simulink model "PCwF2M"  (R2015a)
settings: Solver=ode23  SolverMode=SingleTasking  StartTime=0.0  StopTime=50  RelTol=1e-7
values from neighbouring files (symbols this model uses):
  d1 = 100    [PCwF2Minit.m]
  d2 = 100    [PCwF2Minit.m]
  d3 = 100    [PCwF2Minit.m]
  d4 = 100    [PCwF2Minit.m]
  delta3 = 30    [PCwF2Minit.m]
  delta4 = 30    [PCwF2Minit.m]
  g = [0;0;-9.81]    [PCwF2Minit.m]
  H = blkdiag([eye(3) zeros(3)],[eye(3) zeros(3)])    [PCwF2Minit.m]
  j0 = 10    [PCwF2Minit.m]
  j1 = 10    [PCwF2Minit.m]
  j1d = 1.00*j1    (= 10)    [PCwF2Minit.m]
  j2 = 10    [PCwF2Minit.m]
  j2d = 1.00*j2    (= 10)    [PCwF2Minit.m]
  j3 = 10    [PCwF2Minit.m]
  j3d = 1.00*j3    (= 10)    [PCwF2Minit.m]
  j4 = 10    [PCwF2Minit.m]
  j4d = 1.00*j4    (= 10)    [PCwF2Minit.m]
  k1 = 50    [PCwF2Minit.m]
  k2 = 50    [PCwF2Minit.m]
  k3 = 5    [PCwF2Minit.m]
  k4 = 5    [PCwF2Minit.m]
  kappa3 = 50    [PCwF2Minit.m]
  kappa4 = 50    [PCwF2Minit.m]
  m0 = 10    [PCwF2Minit.m]
  m1 = 10    [PCwF2Minit.m]
  m1d = 1.00*m1    (= 10)    [PCwF2Minit.m]
  m2 = 10    [PCwF2Minit.m]
  m2d = 1.00*m2    (= 10)    [PCwF2Minit.m]
  m3 = 10    [PCwF2Minit.m]
  m3d = 1.00*m3    (= 10)    [PCwF2Minit.m]
  m4 = 10    [PCwF2Minit.m]
  m4d = 1.00*m4    (= 10)    [PCwF2Minit.m]
libraries: aerolibutil x5, dspinverses x3
settings Model: CovSFcnEnable=off  Creator=Martin  LastModifiedBy=mangerer
settings SolverCC: ZeroCrossAlgorithm=Adaptive
settings DataIOCC: LimitDataPoints=off
settings OptimizationCC: BlockReduction=off  BooleanDataType=off
settings DebuggingCC: SaveWithParameterizedLinksMsg=none  UnderspecifiedInitializationDetection=Classic  MergeDetectMultiDrivingBlocksExec=none  SignalResolutionControl=TryResolveAllWithWarning
settings HardwareCC: TargetUnknown=on

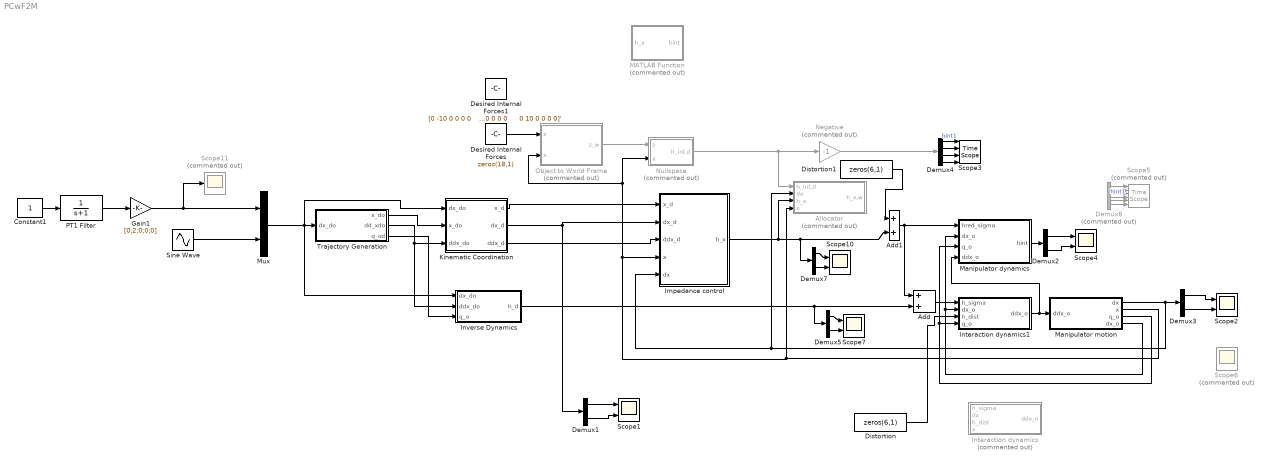
== system PCwF2M ==
  Add : Sum
  Add1 : Sum
  Allocator : Subsystem  Commented=on
  Constant1 : Constant
  Demux{1..3,5,7} (5 alike) : Demux  Outputs=2
  Demux4 : Demux
  Demux6 : Demux  Commented=on  Outputs=6
  Desired Internal Forces : Constant  Value=zeros(18,1)
  Desired Internal Forces1 : Constant  Value="[0 -10 0 0 0 0    10 0 0 0 0 0      0 10 0 0 0 0]'"
  Distortion : Constant  Value=zeros(6,1)
  Distortion1 : Constant  Value=zeros(6,1)
  Gain1 : Gain  Gain=[0;2;0;0;0]
  Impedance control : Subsystem
  Interaction dynamics : Subsystem  Commented=on
  Interaction dynamics1 : Subsystem
  Inverse Dynamics : Subsystem
  Kinematic Coordination : Subsystem
  MATLAB Function : MATLAB Function  Commented=on  TreatAsAtomicUnit=on
  Manipulator dynamics : Subsystem
  Manipulator motion : Subsystem
  Mux : Mux  Inputs=2
  Negative : Gain  Commented=on  Gain=-1
  Nullspace : Subsystem  Commented=on
  Object to World Frame : MATLAB Function  Commented=on  TreatAsAtomicUnit=on
  PT1 Filter : TransferFcn  Denominator=[1 1]
  Scope{1..2,4,7,10} (5 alike) : Scope  NumInputPorts=2
      Scope1 settings: ShowLegends=on  YMin=-1~-1  YMax=1~1
      Scope10 settings: ShowLegends=on  YMin=-75~-75  YMax=75~75  SaveName=ScopeData18
      Scope2 settings: ShowLegends=on  YMin=-0.25~-0.25  YMax=3~3  SaveName=ScopeData2
      Scope4 settings: ShowLegends=on  YMin=-0.2~-0.2  YMax=0.2~0.2  SaveName=ScopeData5
      Scope7 settings: ShowLegends=on  YMin=-75~-75  YMax=75~75  SaveName=ScopeData7
  Scope11 : Scope  Commented=on
      settings: YMin=0.9984  YMax=1  SaveName=ScopeData26
  Scope3 : TimeScope  NumInputPorts=4
  Scope5 : TimeScope  Commented=on  NumInputPorts=6
  Scope6 : Scope  Commented=on  NumInputPorts=4
      settings: ShowLegends=on  YMin=-25~-25~-25~-25  YMax=200~200~200~200  SaveName=ScopeData11
  Sine Wave : Sin  Frequency=2*pi  SampleTime=0
  Trajectory Generation : Subsystem
  wires:
  Manipulator dynamics/1(hint) -> Demux2/1
  Demux2/2 -> Scope4/2
  Demux3/1 -> Scope2/1
  Demux3/2 -> Scope2/2
  Add1/1 -> Manipulator dynamics/1(hred_sigma), Add/1
  Object to World Frame/1(z_w) -> Nullspace/1(z)
  Nullspace/1(h_int,d) -> Negative/1, Allocator/1(h_int,d)
  Demux7/1 -> Scope10/1
  Demux7/2 -> Scope10/2
  PT1 Filter/1 -> Gain1/1
  Gain1/1 -> Mux/1, Scope11/1
  Impedance control/1(h_x) -> Allocator/3(h_x), Add1/2, Demux7/1
  Manipulator motion/1(dx) -> Impedance control/5(dx), Allocator/2(dx), Demux3/1
  Trajectory Generation/2(dd_xdo) -> Inverse Dynamics/2(ddx_do), Kinematic Coordination/3(ddx_do)
  Mux/1 -> Inverse Dynamics/1(dx_do), Kinematic Coordination/1(dx_do), Trajectory Generation/1(dx_do)
  Kinematic Coordination/1(x_d) -> Impedance control/1(x_d)
  Kinematic Coordination/3(ddx_d) -> Impedance control/3(ddx_d)
  Manipulator motion/2(x) -> Object to World Frame/2(x), Nullspace/2(x), Impedance control/4(x), Allocator/4(x)
  Constant1/1 -> PT1 Filter/1
  Demux1/1 -> Scope1/1
  Demux1/2 -> Scope1/2
  Kinematic Coordination/2(dx_d) -> Impedance control/2(dx_d), Demux1/1
  Negative/1 -> Demux4/1
  Demux4/1 -> Scope3/1  "hint1"
  Demux4/2 -> Scope3/2
  Demux4/4 -> Scope3/4
  Sine Wave/1 -> Mux/2
  Demux6/1 -> Scope5/1  "hint1"
  Demux6/2 -> Scope5/2
  Demux6/3 -> Scope5/3
  Demux6/4 -> Scope5/4
  Demux6/5 -> Scope5/5
  Demux6/6 -> Scope5/6
  Demux4/3 -> Scope3/3
  Desired Internal Forces/1 -> Object to World Frame/1(z)
  Add/1 -> Interaction dynamics1/1(h_sigma)
  Interaction dynamics1/1(ddx_o) -> Manipulator dynamics/4(ddx_o), Manipulator motion/1(ddx_o)
  Distortion/1 -> Interaction dynamics1/3(h_dist)
  Manipulator motion/3(q_o) -> Interaction dynamics1/4(q_o), Manipulator dynamics/3(q_o)
  Manipulator motion/4(dx_o) -> Interaction dynamics1/2(dx_o), Manipulator dynamics/2(dx_o)
  Distortion1/1 -> Add1/1
  Demux2/1 -> Scope4/1
  Demux5/1 -> Scope7/1
  Demux5/2 -> Scope7/2
  Inverse Dynamics/1(h_d) -> Demux5/1, Add/2
  Trajectory Generation/1(x_do) -> Kinematic Coordination/2(x_do)
  Trajectory Generation/3(q_od) -> Inverse Dynamics/3(q_o)

== system PCwF2M/Allocator ==
  h_int,d : Inport
  dx : Inport  Port=2
  h_x : Inport  Port=3
  x : Inport  Port=4
  Add : Sum  Inputs=-+
  Add1 : Sum
  Divide : Product  Inputs=*/*  Multiplication=Matrix(*)
  Divide1 : Product  Inputs=*/*  Multiplication=Matrix(*)
  Divide2 : Product  Inputs=*/*  Multiplication=Matrix(*)
  Inertia : Constant  Value=blkdiag(m1d*eye(3), j1d*eye(3), m2d*eye(3), j2d*eye(3), m3d*eye(3), j3d*eye(3), m4d*eye(3), j4d*eye(3))
  MATLAB Function : MATLAB Function  TreatAsAtomicUnit=on
  MATLAB Function1 : MATLAB Function  TreatAsAtomicUnit=on
  Math Function : Math  Operator=transpose  SaturateOnIntegerOverflow=on
  h_x,w : Outport
  wires:
  dx/1 -> MATLAB Function1/1(dx)
  Divide/1 -> h_x,w/1
  Math Function/1 -> Divide1/3, Divide/1
  MATLAB Function/1(Ared) -> Math Function/1, Divide2/1, Divide1/1
  Divide1/1 -> Divide/2
  Inertia/1 -> Divide1/2, Divide2/2
  MATLAB Function1/1(bred) -> Add/2
  Add/1 -> Divide/3
  Divide2/1 -> Add/1
  Add1/1 -> Divide2/3
  h_int,d/1 -> Add1/1
  h_x/1 -> Add1/2
  x/1 -> MATLAB Function1/2(x), MATLAB Function/1(x)

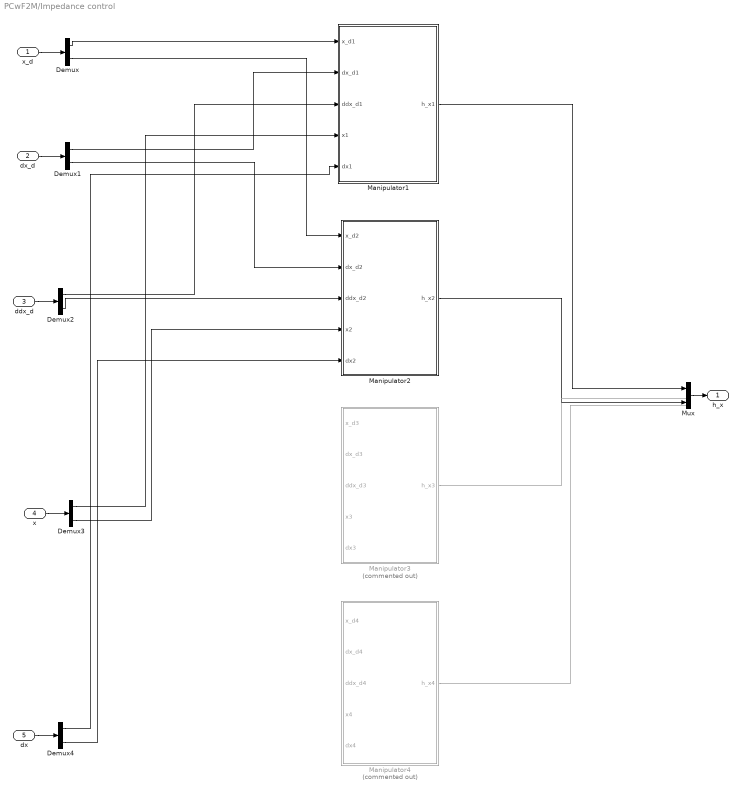
== system PCwF2M/Impedance control ==
  x_d : Inport
  dx_d : Inport  Port=2
  ddx_d : Inport  Port=3
  x : Inport  Port=4
  dx : Inport  Port=5
  Demux{,1..4} (5 alike) : Demux  Outputs=2
  Manipulator1 : Subsystem
  Manipulator2 : Subsystem
  Manipulator3 : Subsystem  Commented=on
  Manipulator4 : Subsystem  Commented=on
  Mux : Mux  Inputs=2
  h_x : Outport
  wires:
  dx/1 -> Demux4/1
  x/1 -> Demux3/1
  ddx_d/1 -> Demux2/1
  dx_d/1 -> Demux1/1
  x_d/1 -> Demux/1
  Demux/1 -> Manipulator1/1(x_d1)
  Demux/2 -> Manipulator2/1(x_d2)
  ? -> Manipulator3/1(x_d3)
  ? -> Manipulator4/1(x_d4)
  Demux1/1 -> Manipulator1/2(dx_d1)
  Demux1/2 -> Manipulator2/2(dx_d2)
  ? -> Manipulator3/2(dx_d3)
  ? -> Manipulator4/2(dx_d4)
  Demux2/1 -> Manipulator1/3(ddx_d1)
  Demux2/2 -> Manipulator2/3(ddx_d2)
  ? -> Manipulator3/3(ddx_d3)
  ? -> Manipulator4/3(ddx_d4)
  Demux3/1 -> Manipulator1/4(x1)
  Demux3/2 -> Manipulator2/4(x2)
  ? -> Manipulator3/4(x3)
  ? -> Manipulator4/4(x4)
  ? -> Manipulator4/5(dx4)
  ? -> Manipulator3/5(dx3)
  Demux4/2 -> Manipulator2/5(dx2)
  Demux4/1 -> Manipulator1/5(dx1)
  Mux/1 -> h_x/1
  Manipulator1/1(h_x1) -> Mux/1
  Manipulator2/1(h_x2) -> Mux/2
  Manipulator3/1(h_x3) -> ?
  Manipulator4/1(h_x4) -> ?

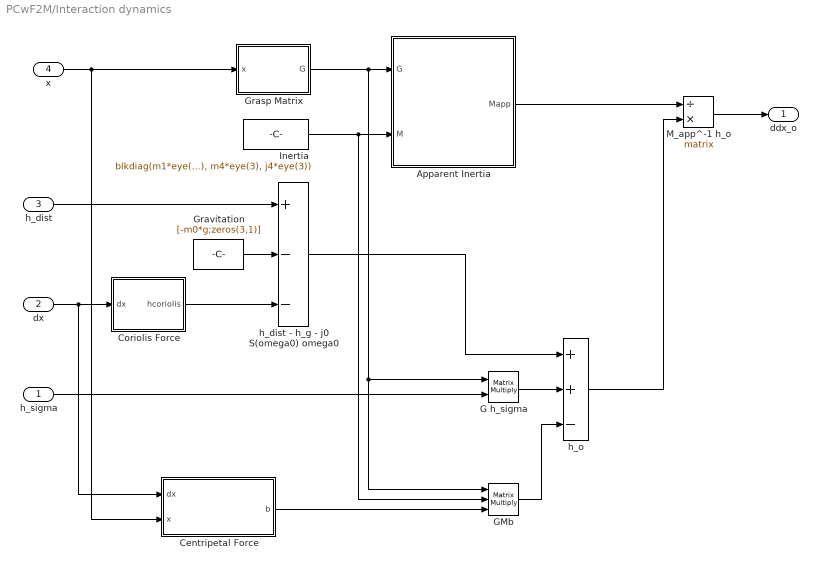
== system PCwF2M/Interaction dynamics ==
  h_sigma : Inport
  dx : Inport  Port=2
  h_dist : Inport  Port=3
  x : Inport  Port=4
  Apparent Inertia : MATLAB Function  TreatAsAtomicUnit=on
  Centripetal Force : MATLAB Function  TreatAsAtomicUnit=on
  Coriolis Force : MATLAB Function  TreatAsAtomicUnit=on
  G h_sigma : Product  Multiplication=Matrix(*)
  GMb : Product  Inputs=***  Multiplication=Matrix(*)
  Grasp Matrix : MATLAB Function  TreatAsAtomicUnit=on
  Gravitation : Constant  Value=[-m0*g;zeros(3,1)]
  Inertia : Constant  Value=blkdiag(m1*eye(3), j1*eye(3), m2*eye(3), j2*eye(3), m3*eye(3), j3*eye(3), m4*eye(3), j4*eye(3))
  M_app^-1 h_o : Product  Inputs=/*  Multiplication=Matrix(*)
  "h_dist - h_g - j0 S(omega0) omega0 " : Sum  Inputs=+--
  h_o : Sum  Inputs=++-
  ddx_o : Outport
  wires:
  Grasp Matrix/1(G) -> G h_sigma/1, GMb/1, Apparent Inertia/1(G)
  Inertia/1 -> GMb/2, Apparent Inertia/2(M)
  Apparent Inertia/1(Mapp) -> M_app^-1 h_o/1
  h_o/1 -> M_app^-1 h_o/2
  G h_sigma/1 -> h_o/2
  h_sigma/1 -> G h_sigma/2
  "h_dist - h_g - j0 S(omega0) omega0 "/1 -> h_o/1
  h_dist/1 -> "h_dist - h_g - j0 S(omega0) omega0 "/1
  Gravitation/1 -> "h_dist - h_g - j0 S(omega0) omega0 "/2
  dx/1 -> Centripetal Force/1(dx), Coriolis Force/1(dx)
  Coriolis Force/1(hcoriolis) -> "h_dist - h_g - j0 S(omega0) omega0 "/3
  GMb/1 -> h_o/3
  Centripetal Force/1(b) -> GMb/3
  M_app^-1 h_o/1 -> ddx_o/1
  x/1 -> Centripetal Force/2(x), Grasp Matrix/1(x)

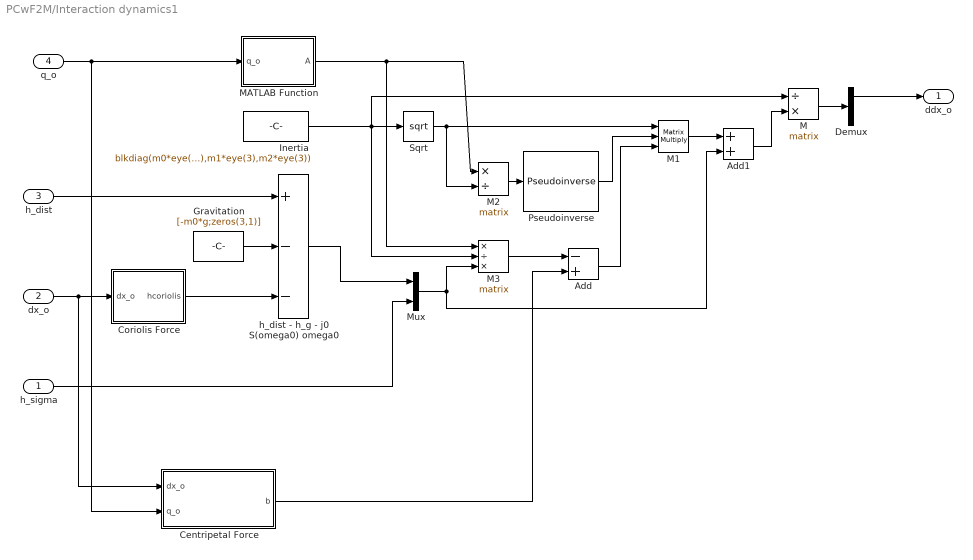
== system PCwF2M/Interaction dynamics1 ==
  h_sigma : Inport
  dx_o : Inport  Port=2
  h_dist : Inport  Port=3
  q_o : Inport  Port=4
  Add : Sum  Inputs=-+
  Add1 : Sum
  Centripetal Force : MATLAB Function  TreatAsAtomicUnit=on
  Coriolis Force : MATLAB Function  TreatAsAtomicUnit=on
  Demux : Demux  Outputs=2
  Gravitation : Constant  Value=[-m0*g;zeros(3,1)]
  Inertia : Constant  Value=blkdiag(m0*eye(3),j0*eye(3),m1*eye(3),m2*eye(3))
  M : Product  Inputs=/*  Multiplication=Matrix(*)
  M1 : Product  Inputs=***  Multiplication=Matrix(*)
  M2 : Product  Inputs=*/  Multiplication=Matrix(*)
  M3 : Product  Inputs=*/*  Multiplication=Matrix(*)
  MATLAB Function : MATLAB Function  TreatAsAtomicUnit=on
  Mux : Mux  Inputs=2
  Pseudoinverse : dspinverses/Pseudoinverse  wanterr=off
  Sqrt : Sqrt  SaturateOnIntegerOverflow=on
  "h_dist - h_g - j0 S(omega0) omega0 " : Sum  Inputs=+--
  ddx_o : Outport
  wires:
  h_dist/1 -> "h_dist - h_g - j0 S(omega0) omega0 "/1
  Gravitation/1 -> "h_dist - h_g - j0 S(omega0) omega0 "/2
  dx_o/1 -> Centripetal Force/1(dx_o), Coriolis Force/1(dx_o)
  Coriolis Force/1(hcoriolis) -> "h_dist - h_g - j0 S(omega0) omega0 "/3
  q_o/1 -> MATLAB Function/1(q_o), Centripetal Force/2(q_o)
  Inertia/1 -> M/1, M3/2, Sqrt/1
  Sqrt/1 -> M2/2, M1/1
  MATLAB Function/1(A) -> M3/1, M2/1
  M2/1 -> Pseudoinverse/1
  Pseudoinverse/1 -> M1/2
  Add/1 -> M1/3
  Centripetal Force/1(b) -> Add/2
  M3/1 -> Add/1
  Mux/1 -> Add1/2, M3/3
  "h_dist - h_g - j0 S(omega0) omega0 "/1 -> Mux/1
  h_sigma/1 -> Mux/2
  M/1 -> Demux/1
  Demux/1 -> ddx_o/1
  M1/1 -> Add1/1
  Add1/1 -> M/2

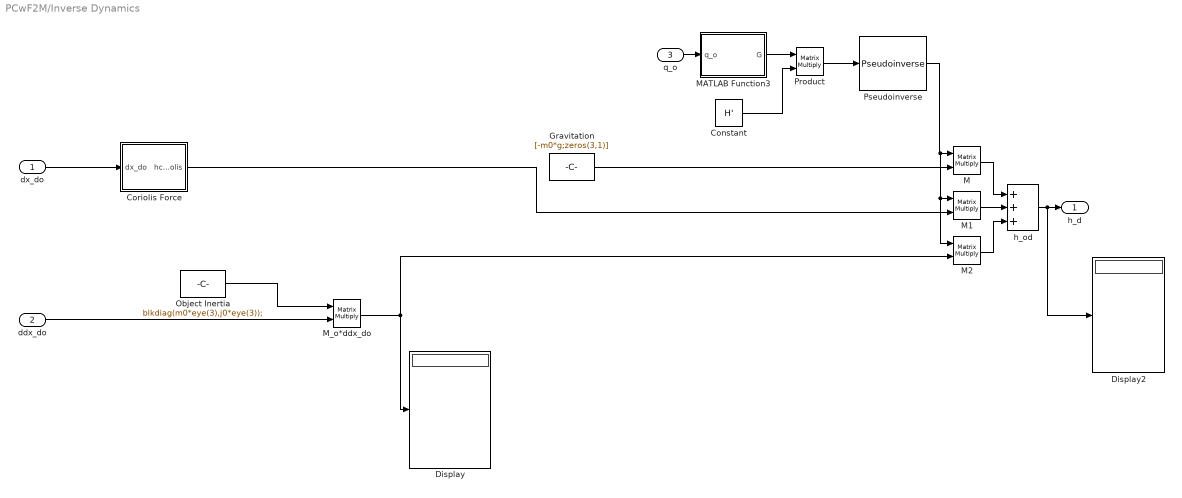
== system PCwF2M/Inverse Dynamics ==
  dx_do : Inport
  ddx_do : Inport  Port=2
  q_o : Inport  Port=3
  Constant : Constant  Value=H'
  Coriolis Force : MATLAB Function  TreatAsAtomicUnit=on
  Display : Display
  Display2 : Display
  Gravitation : Constant  Value=[-m0*g;zeros(3,1)]
  M : Product  Multiplication=Matrix(*)
  M1 : Product  Multiplication=Matrix(*)
  M2 : Product  Multiplication=Matrix(*)
  MATLAB Function3 : MATLAB Function  TreatAsAtomicUnit=on
  M_o*ddx_do : Product  Multiplication=Matrix(*)
  Object Inertia : Constant  Value=blkdiag(m0*eye(3),j0*eye(3));
  Product : Product  Multiplication=Matrix(*)
  Pseudoinverse : dspinverses/Pseudoinverse  wanterr=off
  h_od : Sum  Inputs=+++
  h_d : Outport
  wires:
  ddx_do/1 -> M_o*ddx_do/2
  Object Inertia/1 -> M_o*ddx_do/1
  dx_do/1 -> Coriolis Force/1(dx_do)
  q_o/1 -> MATLAB Function3/1(q_o)
  M_o*ddx_do/1 -> Display/1, M2/2
  Coriolis Force/1(hcoriolis) -> M1/2
  Pseudoinverse/1 -> M2/1, M1/1, M/1
  MATLAB Function3/1(G) -> Product/1
  Product/1 -> Pseudoinverse/1
  Constant/1 -> Product/2
  M1/1 -> h_od/2
  M/1 -> h_od/1
  M2/1 -> h_od/3
  h_od/1 -> Display2/1, h_d/1
  Gravitation/1 -> M/2

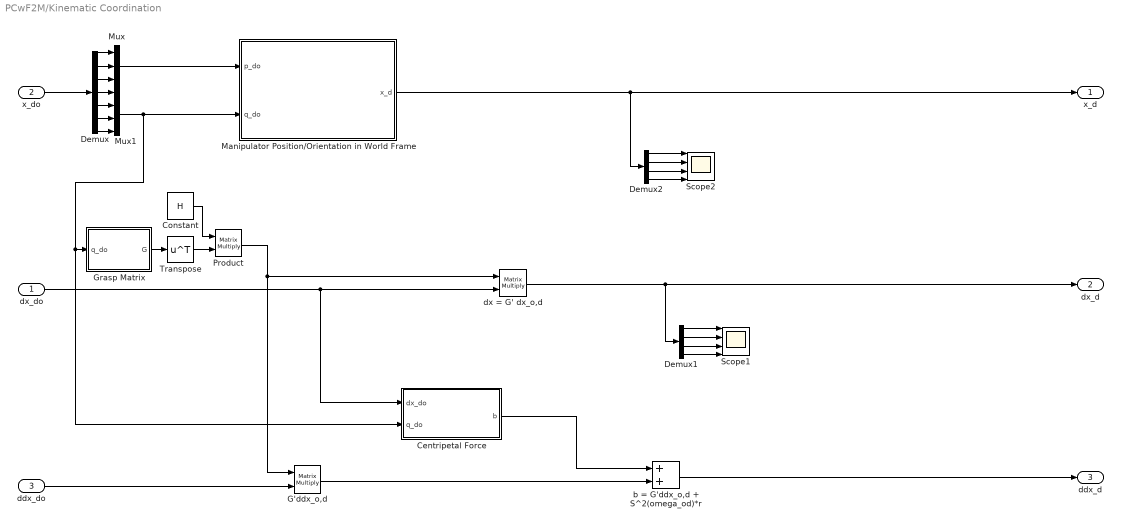
== system PCwF2M/Kinematic Coordination ==
  dx_do : Inport
  x_do : Inport  Port=2
  ddx_do : Inport  Port=3
  Centripetal Force : MATLAB Function  TreatAsAtomicUnit=on
  Constant : Constant  Value=H
  Demux : Demux  Outputs=7
  Demux1 : Demux
  Demux2 : Demux
  G'ddx_o,d : Product  Multiplication=Matrix(*)
  Grasp Matrix : MATLAB Function  TreatAsAtomicUnit=on
  Manipulator Position/Orientation in World Frame : MATLAB Function  TreatAsAtomicUnit=on
  Mux : Mux  Inputs=3
  Mux1 : Mux
  Product : Product  Multiplication=Matrix(*)
  Scope1 : Scope  NumInputPorts=4
      settings: ShowLegends=on  YMin=-1.5~-1.5~-1.5~-1.5  YMax=6~5.5~6~5.5  SaveName=ScopeData3
  Scope2 : Scope  NumInputPorts=4
      settings: ShowLegends=on  YMin=-1.5~-1.5~-1.5~-1.5  YMax=6~5.5~6~5.5  SaveName=ScopeData4
  Transpose : Math  Operator=transpose  SaturateOnIntegerOverflow=on
  b = G'ddx_o,d + S^2(omega_od)*r : Sum
  dx = G' dx_o,d : Product  Multiplication=Matrix(*)
  x_d : Outport
  dx_d : Outport  Port=2
  ddx_d : Outport  Port=3
  wires:
  Grasp Matrix/1(G) -> Transpose/1
  dx = G' dx_o,d/1 -> Demux1/1, dx_d/1
  x_do/1 -> Demux/1
  Demux/1 -> Mux/1
  Demux/2 -> Mux/2
  Demux/3 -> Mux/3
  Demux/5 -> Mux1/2
  Demux/6 -> Mux1/3
  Demux/7 -> Mux1/4
  Demux/4 -> Mux1/1
  Mux/1 -> Manipulator Position/Orientation in World Frame/1(p_do)
  Centripetal Force/1(b) -> b = G'ddx_o,d + S^2(omega_od)*r/1
  ddx_do/1 -> G'ddx_o,d/2
  G'ddx_o,d/1 -> b = G'ddx_o,d + S^2(omega_od)*r/2
  b = G'ddx_o,d + S^2(omega_od)*r/1 -> ddx_d/1
  dx_do/1 -> Centripetal Force/1(dx_do), dx = G' dx_o,d/2
  Demux1/1 -> Scope1/1
  Demux1/2 -> Scope1/2
  Demux1/3 -> Scope1/3
  Demux1/4 -> Scope1/4
  Manipulator Position/Orientation in World Frame/1(x_d) -> Demux2/1, x_d/1
  Demux2/1 -> Scope2/1
  Demux2/2 -> Scope2/2
  Demux2/3 -> Scope2/3
  Demux2/4 -> Scope2/4
  Transpose/1 -> Product/2
  Product/1 -> dx = G' dx_o,d/1, G'ddx_o,d/1
  Constant/1 -> Product/1
  Mux1/1 -> Centripetal Force/2(q_do), Grasp Matrix/1(q_do), Manipulator Position/Orientation in World Frame/2(q_do)

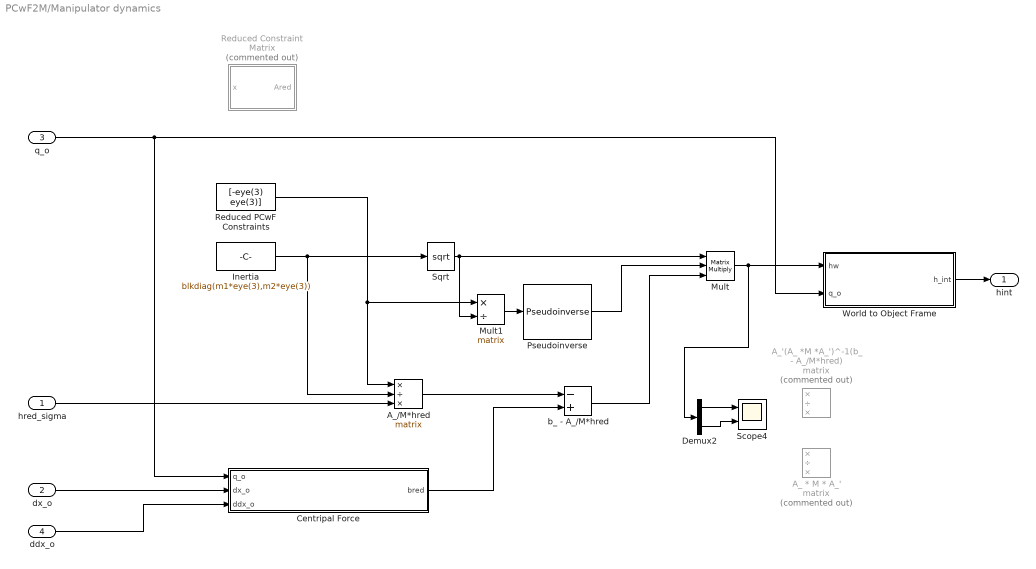
== system PCwF2M/Manipulator dynamics ==
  hred_sigma : Inport
  dx_o : Inport  Port=2
  q_o : Inport  Port=3
  ddx_o : Inport  Port=4
  A_ * M * A_' : Product  Commented=on  Inputs=*/*  Multiplication=Matrix(*)
  A_'(A_ *M *A_')^-1(b_ - A_/M*hred) : Product  Commented=on  Inputs=*/*  Multiplication=Matrix(*)
  A_/M*hred : Product  Inputs=*/*  Multiplication=Matrix(*)
  Centripal Force : MATLAB Function  TreatAsAtomicUnit=on
  Demux2 : Demux  Outputs=2
  Inertia : Constant  Value=blkdiag(m1*eye(3),m2*eye(3))
  Mult : Product  Inputs=***  Multiplication=Matrix(*)
  Mult1 : Product  Inputs=*/  Multiplication=Matrix(*)
  Pseudoinverse : dspinverses/Pseudoinverse  wanterr=off
  Reduced Constraint Matrix : MATLAB Function  Commented=on  TreatAsAtomicUnit=on
  Reduced PCwF Constraints : Constant  Value=[-eye(3) eye(3)]
  Scope4 : Scope  NumInputPorts=2
      settings: ShowLegends=on  YMin=-0.2~-0.175  YMax=0.175~0.2  SaveName=ScopeData8
  Sqrt : Sqrt  SaturateOnIntegerOverflow=on
  World to Object Frame : MATLAB Function  TreatAsAtomicUnit=on
  b_ - A_/M*hred : Sum  Inputs=-+
  hint : Outport
  wires:
  Inertia/1 -> Sqrt/1, A_/M*hred/2
  A_/M*hred/1 -> b_ - A_/M*hred/1
  hred_sigma/1 -> A_/M*hred/3
  World to Object Frame/1(h_int) -> hint/1
  q_o/1 -> Centripal Force/1(q_o), World to Object Frame/2(q_o)
  Centripal Force/1(bred) -> b_ - A_/M*hred/2
  b_ - A_/M*hred/1 -> Mult/3
  Sqrt/1 -> Mult1/2, Mult/1
  Mult1/1 -> Pseudoinverse/1
  Pseudoinverse/1 -> Mult/2
  Reduced PCwF Constraints/1 -> A_/M*hred/1, Mult1/1
  dx_o/1 -> Centripal Force/2(dx_o)
  ddx_o/1 -> Centripal Force/3(ddx_o)
  Mult/1 -> Demux2/1, World to Object Frame/1(hw)
  Demux2/2 -> Scope4/2
  Demux2/1 -> Scope4/1

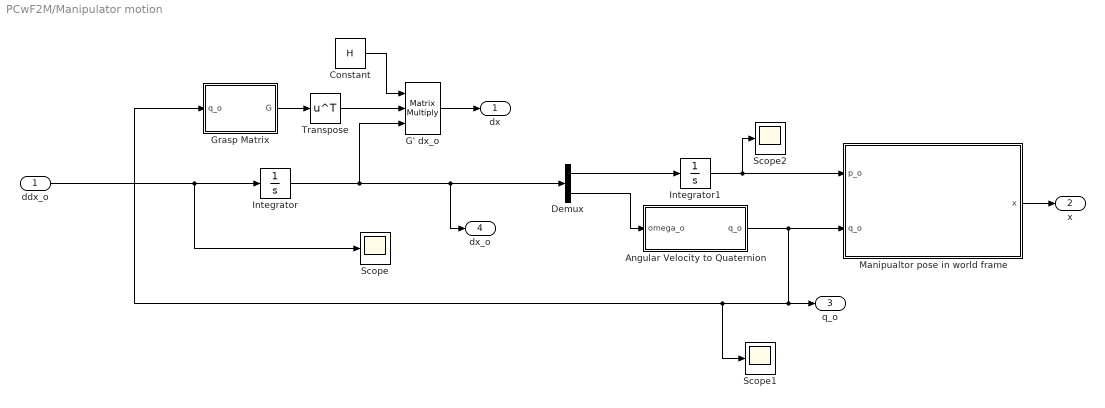
== system PCwF2M/Manipulator motion ==
  ddx_o : Inport
  Angular Velocity to Quaternion : Subsystem
  Constant : Constant  Value=H
  Demux : Demux  Outputs=2
  G' dx_o : Product  Inputs=3  Multiplication=Matrix(*)
  Grasp Matrix : MATLAB Function  TreatAsAtomicUnit=on
  Integrator : Integrator  InitialCondition=zeros(6,1)
  Integrator1 : Integrator  InitialCondition=[0 0 0]'
  Manipualtor pose in world frame : MATLAB Function  TreatAsAtomicUnit=on
  Scope : Scope
      settings: ShowLegends=on  YMin=-3.5  YMax=3.5  SaveName=ScopeData14
  Scope1 : Scope
      settings: YMin=-0.5  YMax=1  SaveName=ScopeData12
  Scope2 : Scope
      settings: ShowLegends=on  YMin=-10  YMax=150  SaveName=ScopeData6
  Transpose : Math  Operator=transpose  SaturateOnIntegerOverflow=on
  dx : Outport
  x : Outport  Port=2
  q_o : Outport  Port=3
  dx_o : Outport  Port=4
  wires:
  ddx_o/1 -> Scope/1, Integrator/1
  Integrator/1 -> G' dx_o/3, dx_o/1, Demux/1
  Grasp Matrix/1(G) -> Transpose/1
  G' dx_o/1 -> dx/1
  Demux/2 -> Angular Velocity to Quaternion/1(omega_o)
  Demux/1 -> Integrator1/1
  Integrator1/1 -> Scope2/1, Manipualtor pose in world frame/1(p_o)
  Manipualtor pose in world frame/1(x) -> x/1
  Angular Velocity to Quaternion/1(q_o) -> Scope1/1, Grasp Matrix/1(q_o), q_o/1, Manipualtor pose in world frame/2(q_o)
  Transpose/1 -> G' dx_o/2
  Constant/1 -> G' dx_o/1

== system PCwF2M/Nullspace ==
  z : Inport
  x : Inport  Port=2
  A_' * z : Product  Multiplication=Matrix(*)
  Reduced Constraint Matrix : MATLAB Function  TreatAsAtomicUnit=on
  Transpose : Math  Operator=transpose  SaturateOnIntegerOverflow=on
  h_int,d : Outport
  wires:
  Reduced Constraint Matrix/1(Ared) -> Transpose/1
  Transpose/1 -> A_' * z/1
  z/1 -> A_' * z/2
  A_' * z/1 -> h_int,d/1
  x/1 -> Reduced Constraint Matrix/1(x)

== system PCwF2M/Trajectory Generation ==
  dx_do : Inport
  Angular Velocity to Quaternion Orientation : Subsystem
  Demux : Demux  Outputs=2
  Demux1 : Demux  Outputs=7
  Derivative : Derivative
  Integrator : Integrator  InitialCondition=zeros(3,1)
  Mux : Mux  Inputs=2
  Mux1 : Mux  Inputs=3
  Mux2 : Mux
  Mux3 : Mux  Inputs=2
  Quaternion Normalize : aerolibutil/Quaternion Normalize
  x_do : Outport
  dd_xdo : Outport  Port=2
  q_od : Outport  Port=3
  wires:
  dx_do/1 -> Derivative/1, Demux/1
  Demux/2 -> Angular Velocity to Quaternion Orientation/1(omega_do)
  Demux/1 -> Integrator/1
  Angular Velocity to Quaternion Orientation/1(q_do) -> Quaternion Normalize/1
  Integrator/1 -> Mux/1
  Derivative/1 -> dd_xdo/1
  Quaternion Normalize/1 -> Mux/2
  Demux1/1 -> Mux1/1
  Demux1/2 -> Mux1/2
  Demux1/3 -> Mux1/3
  Demux1/4 -> Mux2/1
  Demux1/5 -> Mux2/2
  Demux1/6 -> Mux2/3
  Demux1/7 -> Mux2/4
  Mux/1 -> Demux1/1
  Mux1/1 -> Mux3/1
  Mux3/1 -> x_do/1
  Mux2/1 -> q_od/1, Mux3/2

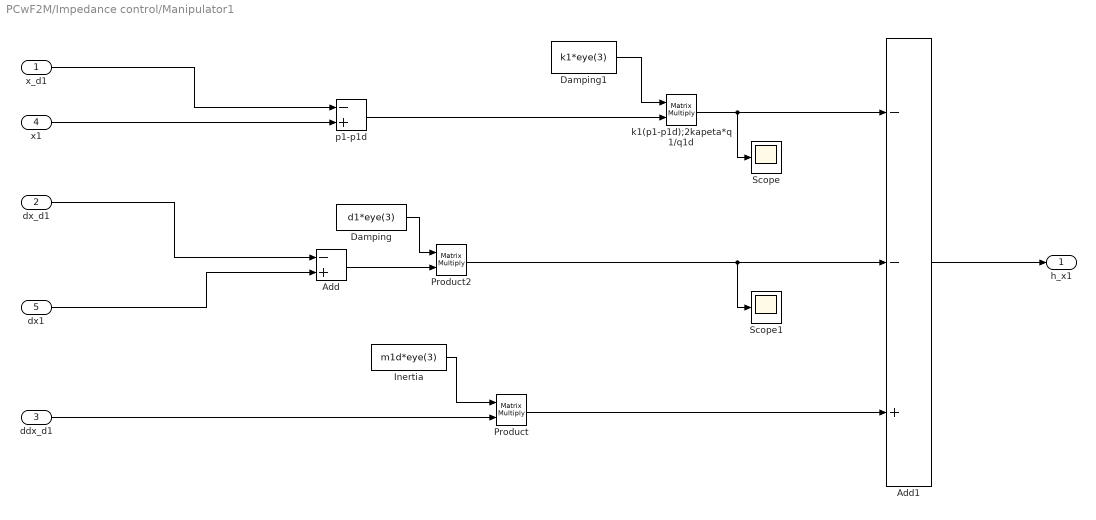
== system PCwF2M/Impedance control/Manipulator1 ==
  x_d1 : Inport
  dx_d1 : Inport  Port=2
  ddx_d1 : Inport  Port=3
  x1 : Inport  Port=4
  dx1 : Inport  Port=5
  Add : Sum  Inputs=-+
  Add1 : Sum  Inputs=--+
  Damping : Constant  Value=d1*eye(3)
  Damping1 : Constant  Value=k1*eye(3)
  Inertia : Constant  Value=m1d*eye(3)
  Product : Product  Multiplication=Matrix(*)
  Product2 : Product  Multiplication=Matrix(*)
  Scope : Scope
      settings: TimeRange=200  YMin=-50  YMax=125  SaveName=ScopeData13
  Scope1 : Scope
      settings: TimeRange=200  YMin=-50  YMax=125  SaveName=ScopeData19
  k1(p1-p1d);2kapeta*q1/q1d : Product  Multiplication=Matrix(*)
  p1-p1d : Sum  Inputs=-+
  h_x1 : Outport
  wires:
  Add/1 -> Product2/2
  Damping/1 -> Product2/1
  dx_d1/1 -> Add/1
  dx1/1 -> Add/2
  Inertia/1 -> Product/1
  Add1/1 -> h_x1/1
  k1(p1-p1d);2kapeta*q1/q1d/1 -> Scope/1, Add1/1
  Product2/1 -> Scope1/1, Add1/2
  Product/1 -> Add1/3
  ddx_d1/1 -> Product/2
  Damping1/1 -> k1(p1-p1d);2kapeta*q1/q1d/1
  p1-p1d/1 -> k1(p1-p1d);2kapeta*q1/q1d/2
  x_d1/1 -> p1-p1d/1
  x1/1 -> p1-p1d/2

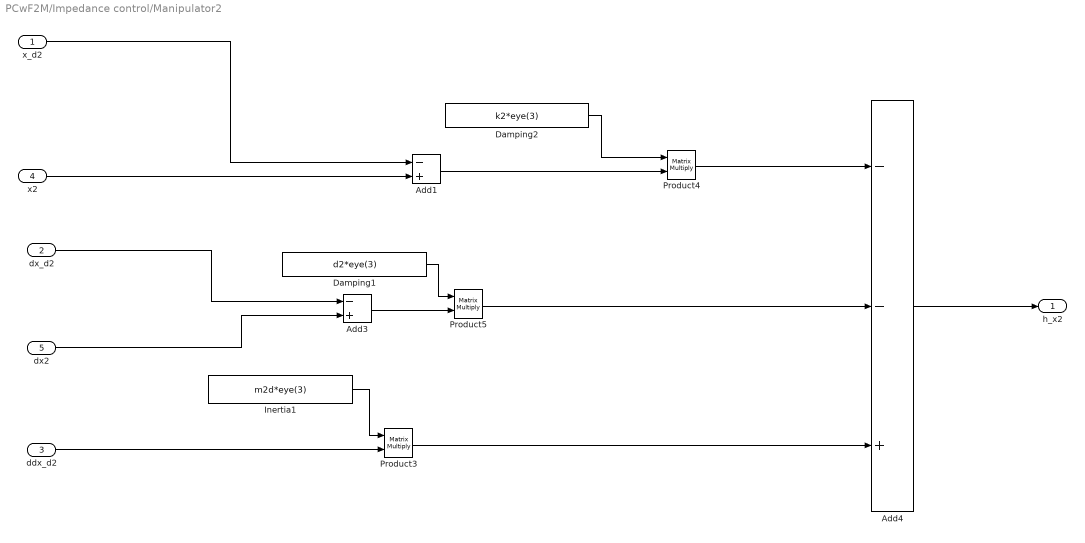
== system PCwF2M/Impedance control/Manipulator2 ==
  x_d2 : Inport
  dx_d2 : Inport  Port=2
  ddx_d2 : Inport  Port=3
  x2 : Inport  Port=4
  dx2 : Inport  Port=5
  Add1 : Sum  Inputs=-+
  Add3 : Sum  Inputs=-+
  Add4 : Sum  Inputs=--+
  Damping1 : Constant  Value=d2*eye(3)
  Damping2 : Constant  Value=k2*eye(3)
  Inertia1 : Constant  Value=m2d*eye(3)
  Product3 : Product  Multiplication=Matrix(*)
  Product4 : Product  Multiplication=Matrix(*)
  Product5 : Product  Multiplication=Matrix(*)
  h_x2 : Outport
  wires:
  Add3/1 -> Product5/2
  Damping1/1 -> Product5/1
  dx_d2/1 -> Add3/1
  dx2/1 -> Add3/2
  Inertia1/1 -> Product3/1
  Add4/1 -> h_x2/1
  Product4/1 -> Add4/1
  Product5/1 -> Add4/2
  Product3/1 -> Add4/3
  ddx_d2/1 -> Product3/2
  Damping2/1 -> Product4/1
  x_d2/1 -> Add1/1
  Add1/1 -> Product4/2
  x2/1 -> Add1/2

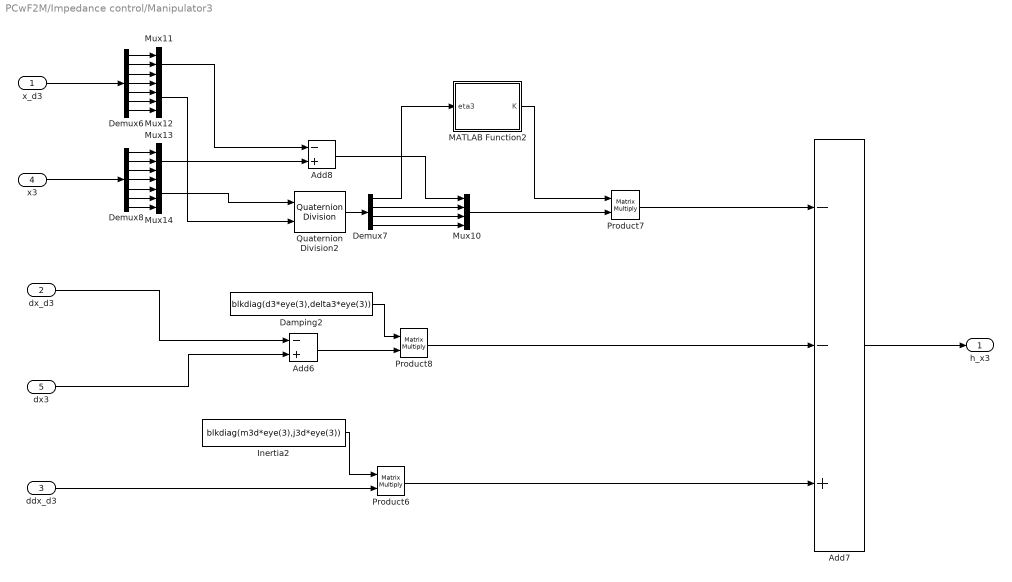
== system PCwF2M/Impedance control/Manipulator3 ==
  x_d3 : Inport
  dx_d3 : Inport  Port=2
  ddx_d3 : Inport  Port=3
  x3 : Inport  Port=4
  dx3 : Inport  Port=5
  Add6 : Sum  Inputs=-+
  Add7 : Sum  Inputs=--+
  Add8 : Sum  Inputs=-+
  Damping2 : Constant  Value=blkdiag(d3*eye(3),delta3*eye(3))
  Demux6 : Demux  Outputs=7
  Demux7 : Demux
  Demux8 : Demux  Outputs=7
  Inertia2 : Constant  Value=blkdiag(m3d*eye(3),j3d*eye(3))
  MATLAB Function2 : MATLAB Function  TreatAsAtomicUnit=on
  Mux10 : Mux
  Mux11 : Mux  Inputs=3
  Mux12 : Mux
  Mux13 : Mux  Inputs=3
  Mux14 : Mux
  Product6 : Product  Multiplication=Matrix(*)
  Product7 : Product  Multiplication=Matrix(*)
  Product8 : Product  Multiplication=Matrix(*)
  Quaternion Division2 : aerolibutil/Quaternion Division
  h_x3 : Outport
  wires:
  Add6/1 -> Product8/2
  Damping2/1 -> Product8/1
  dx_d3/1 -> Add6/1
  dx3/1 -> Add6/2
  MATLAB Function2/1(K) -> Product7/1
  Demux7/1 -> MATLAB Function2/1(eta3)
  Add8/1 -> Mux10/1
  Demux7/2 -> Mux10/2
  Demux7/3 -> Mux10/3
  Demux7/4 -> Mux10/4
  x3/1 -> Demux8/1
  x_d3/1 -> Demux6/1
  Demux6/2 -> Mux11/2
  Demux6/1 -> Mux11/1
  Demux6/3 -> Mux11/3
  Demux6/4 -> Mux12/1
  Demux6/5 -> Mux12/2
  Demux6/6 -> Mux12/3
  Demux6/7 -> Mux12/4
  Demux8/2 -> Mux13/2
  Demux8/1 -> Mux13/1
  Demux8/3 -> Mux13/3
  Demux8/4 -> Mux14/1
  Demux8/5 -> Mux14/2
  Demux8/6 -> Mux14/3
  Demux8/7 -> Mux14/4
  Mux11/1 -> Add8/1
  Mux13/1 -> Add8/2
  Quaternion Division2/1 -> Demux7/1
  Mux10/1 -> Product7/2
  Inertia2/1 -> Product6/1
  Add7/1 -> h_x3/1
  Product7/1 -> Add7/1
  Product8/1 -> Add7/2
  Product6/1 -> Add7/3
  ddx_d3/1 -> Product6/2
  Mux14/1 -> Quaternion Division2/1
  Mux12/1 -> Quaternion Division2/2

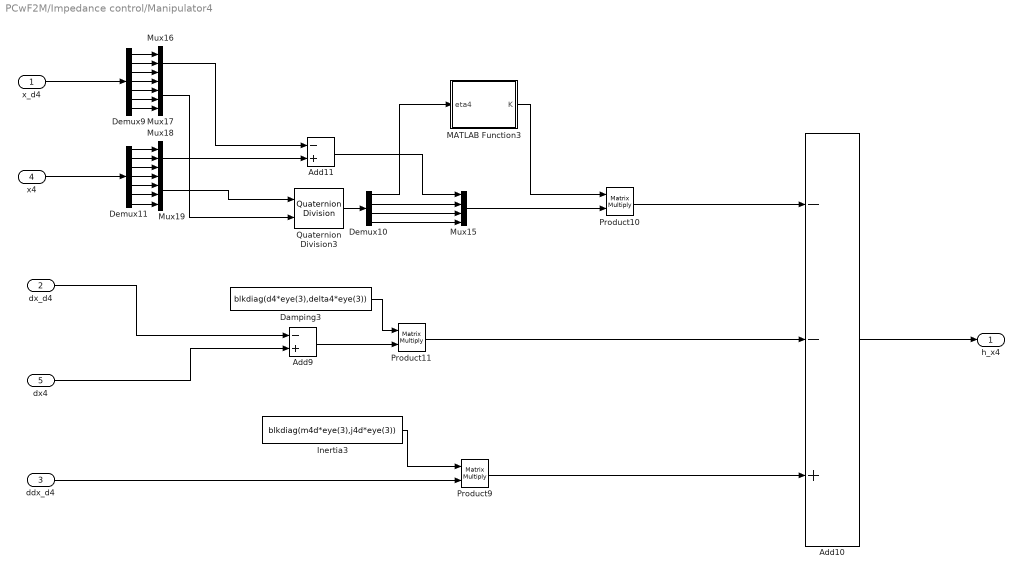
== system PCwF2M/Impedance control/Manipulator4 ==
  x_d4 : Inport
  dx_d4 : Inport  Port=2
  ddx_d4 : Inport  Port=3
  x4 : Inport  Port=4
  dx4 : Inport  Port=5
  Add10 : Sum  Inputs=--+
  Add11 : Sum  Inputs=-+
  Add9 : Sum  Inputs=-+
  Damping3 : Constant  Value=blkdiag(d4*eye(3),delta4*eye(3))
  Demux10 : Demux
  Demux11 : Demux  Outputs=7
  Demux9 : Demux  Outputs=7
  Inertia3 : Constant  Value=blkdiag(m4d*eye(3),j4d*eye(3))
  MATLAB Function3 : MATLAB Function  TreatAsAtomicUnit=on
  Mux15 : Mux
  Mux16 : Mux  Inputs=3
  Mux17 : Mux
  Mux18 : Mux  Inputs=3
  Mux19 : Mux
  Product10 : Product  Multiplication=Matrix(*)
  Product11 : Product  Multiplication=Matrix(*)
  Product9 : Product  Multiplication=Matrix(*)
  Quaternion Division3 : aerolibutil/Quaternion Division
  h_x4 : Outport
  wires:
  Add9/1 -> Product11/2
  Damping3/1 -> Product11/1
  dx_d4/1 -> Add9/1
  dx4/1 -> Add9/2
  MATLAB Function3/1(K) -> Product10/1
  Demux10/1 -> MATLAB Function3/1(eta4)
  Add11/1 -> Mux15/1
  Demux10/2 -> Mux15/2
  Demux10/3 -> Mux15/3
  Demux10/4 -> Mux15/4
  x4/1 -> Demux11/1
  x_d4/1 -> Demux9/1
  Demux9/2 -> Mux16/2
  Demux9/1 -> Mux16/1
  Demux9/3 -> Mux16/3
  Demux9/4 -> Mux17/1
  Demux9/5 -> Mux17/2
  Demux9/6 -> Mux17/3
  Demux9/7 -> Mux17/4
  Demux11/2 -> Mux18/2
  Demux11/1 -> Mux18/1
  Demux11/3 -> Mux18/3
  Demux11/4 -> Mux19/1
  Demux11/5 -> Mux19/2
  Demux11/6 -> Mux19/3
  Demux11/7 -> Mux19/4
  Mux16/1 -> Add11/1
  Mux18/1 -> Add11/2
  Quaternion Division3/1 -> Demux10/1
  Mux15/1 -> Product10/2
  Inertia3/1 -> Product9/1
  Add10/1 -> h_x4/1
  Product10/1 -> Add10/1
  Product11/1 -> Add10/2
  Product9/1 -> Add10/3
  ddx_d4/1 -> Product9/2
  Mux19/1 -> Quaternion Division3/1
  Mux17/1 -> Quaternion Division3/2

== system PCwF2M/Manipulator motion/Angular Velocity to Quaternion ==
  omega_o : Inport
  Constant : Constant  Value=0
  Gain : Gain  Gain=0.5
  Integrator : Integrator  InitialCondition=[1; 0; 0; 0]
  Mux : Mux  Inputs=2
  Quaternion Multiplication : aerolibutil/Quaternion Multiplication
  Scope : Scope
      settings: ShowLegends=on  SaveName=ScopeData9
  q_o : Outport
  wires:
  omega_o/1 -> Gain/1
  Gain/1 -> Mux/2
  Constant/1 -> Mux/1
  Quaternion Multiplication/1 -> Integrator/1
  Integrator/1 -> Quaternion Multiplication/2, q_o/1, Scope/1
  Mux/1 -> Quaternion Multiplication/1

== system PCwF2M/Trajectory Generation/Angular Velocity to Quaternion Orientation ==
  omega_do : Inport
  Constant : Constant  Value=0
  Gain : Gain  Gain=0.5
  Integrator : Integrator  InitialCondition=[1; 0; 0; 0]
  Mux : Mux  Inputs=2
  Quaternion Multiplication : aerolibutil/Quaternion Multiplication
  Scope : Scope
      settings: ShowLegends=on  SaveName=ScopeData9
  q_do : Outport
  wires:
  omega_do/1 -> Gain/1
  Gain/1 -> Mux/2
  Constant/1 -> Mux/1
  Quaternion Multiplication/1 -> Integrator/1
  Integrator/1 -> Quaternion Multiplication/2, Scope/1, q_do/1
  Mux/1 -> Quaternion Multiplication/1

== matlab function PCwF2M/Inverse Dynamics/Coriolis Force ==
  data: dx_do input; hcoriolis output; j0 parameter; m0 parameter
function hcoriolis = CoriolisForce(dx_do,j0,m0)
hcoriolis = [m0*skew_sm(dx_do(4:6))*dx_do(1:3);
        j0*skew_sm(dx_do(4:6))*dx_do(4:6)];

== matlab function PCwF2M/Interaction dynamics1/MATLAB Function ==
  data: r parameter; A output; q_o input
function A = ConstraintMatrix(r,q_o)
% A = [-eye(3) skew_sm(quatrot(x(4:7),r(1:3))) eye(3) zeros(3,21);
%         zeros(3) -eye(3) zeros(3) eye(3) zeros(3,18);
%         -eye(3) skew_sm(quatrot(x(4:7),r(4:6))) zeros(3,6) eye(3) zeros(3,15);
%         zeros(3) -eye(3) zeros(3,9) eye(3) zeros(3,12);
%         -eye(3) skew_sm(quatrot(x(4:7),r(7:9))) zeros(3,12) eye(3) zeros(3,9);
%         zeros(3) -eye(3) zeros(3,15) eye(3) zeros(3,6);
%         -eye(3) skew_sm(quatrot(x(4:7),r(10:12))) zeros(3,18) eye(3) zeros(3);
%         zeros(3) -eye(3) zeros(3,21) eye(3)];
A = [-eye(3) skew_sm(quatrot(q_o,r(1:3))) eye(3) zeros(3);
     -eye(3) skew_sm(quatrot(q_o,r(4:6))) zeros(3) eye(3)];

== matlab function PCwF2M/Interaction dynamics1/Centripetal Force ==
  data: dx_o input; b output; r parameter; q_o input
function b = centripetalforce(dx_o,r,q_o)
b = [skew_sm(dx_o(4:6))*skew_sm(dx_o(4:6))*quatrot(q_o,r(1:3));
     %zeros(3,1);
     skew_sm(dx_o(4:6))*skew_sm(dx_o(4:6))*quatrot(q_o,r(4:6))];
     %zeros(3,1);
%      skew_sm(dx(4:6))*skew_sm(dx(4:6))*quatrot(x(4:7),r(7:9));
%      zeros(3,1);
%      skew_sm(dx(4:6))*skew_sm(dx(4:6))*quatrot(x(4:7),r(10:12));
%      zeros(3,1)];

== matlab function PCwF2M/Interaction dynamics1/Coriolis Force ==
  data: dx_o input; hcoriolis output; j0 parameter; m0 parameter
function hcoriolis = CoriolisForce(dx_o,j0,m0)
hcoriolis = [m0*skew_sm(dx_o(4:6))*dx_o(1:3);
        j0*skew_sm(dx_o(4:6))*dx_o(4:6)];

== matlab function PCwF2M/MATLAB Function ==
  data: h_x input; hint output
function hint = InternalForceOpt(h_x)

%External forces: World to object frame
h_xobj = [quatrot(quatconj(x(4:7)')',h_x(1:3));
         h_x(4:6);
         quatrot(quatconj(x(4:7)')',h_x(7:9));
         h_x(10:12);
         quatrot(quatconj(x(4:7)')',h_X(13:15));
         h_x(16:18);
         quatrot(quatconj(x(4:7)')',h_X(19:21));
         h_x(22:24)];
     
%Coordinate Transformation: Object to contact normal frame
%Contact normals
n_obj = r; %Normals in object frame: same direction than virtual stick of contact points
n_con = [0 0 1]';
%Calculation of rotation matrix based on normal in object and contact frame
% Rn = zeros(12,3);
% for i=0:3
%     v = skew_sm(skew_sm(n_con)*n_obj(3*i+1:3*i+3));
%     Rn(3*i+1:3*i+3,1:3) = eye(3) + v + v*v*(1 -n_con*n_obj(3*i+1:3*i+3))/abs(v);
% end
% Quaternion representation of rotation between two vectors: AxisAngle
q = zeros(16);
k = zeros(4);
for i=0:3
    k(i+1) = skew_sm(n_obj(i*3+1:i*3+3))*n_con;
    q(i*4+2:i*4+4) = k(i+1);
    q(i*4+1) = n_obj(i*3+1:i*3+3)'*n_con;
end


% Simplified AxisAngle to Quaternion

%Sum of external and internal forces in object frame
Ared = [-eye(3) skew_sm(r(4:6)-r(1:3)) eye(3) zeros(3,15);
        -eye(3) skew_sm(r(7:9)-r(1:3)) zeros(3,6) eye(3) zeros(3,9);
        -eye(3) skew_sm(r(10:12)-r(1:3)) zeros(3,12) eye(3) zeros(3)];

cvx_begin %Call convex optimizer
variable z(9) %Declare z to optimize

%Convert total forces in contact normal frame    
h_obj = h_xobj + Ared'*z;

h_con = zeros(24);
for i=0:3
    h_con(6*i+1:6*i+3) = quatrot(q(4*i+1:4*i+4,h_obj(6*i+1:6*i+3));
    h_con(6*i+4:6*i+6) =  h_obj(6*i+4:6*i+6);
end

S1 = [0 0 1; 0 0 0; 1 0 0; 0 0 0; 0 0 1; 0 1 0; mu*eye(3)];
S2 = [0 0 1; 0 0 0; 1 0 0; 0 0 0; 0 0 1; 0 1 0; mu*eye(3)];
S3 = [0 0 1; 0 0 0; 1 0 0; 0 0 0; 0 0 1; 0 1 0; mu*eye(3)];
S4 = [0 0 1; 0 0 0; 1 0 0; 0 0 0; 0 0 1; 0 1 0; mu*eye(3)];

== matlab function PCwF2M/Kinematic Coordination/Grasp Matrix ==
  data: r parameter; G output; q_do input
function G = GraspMatrix(r,q_do)
% G = [eye(3) zeros(3) eye(3) zeros(3) eye(3) zeros(3) eye(3) zeros(3);
%     skew_sm(quatrot(x(4:7),r(1:3))) eye(3) skew_sm(quatrot(x(4:7),r(4:6))) eye(3) skew_sm(quatrot(x(4:7),r(7:9))) eye(3) skew_sm(quatrot(x(4:7),r(10:12))) eye(3)];
 G = [eye(3) zeros(3) eye(3) zeros(3);
   skew_sm(quatrot(q_do,r(1:3))) eye(3) skew_sm(quatrot(q_do,r(4:6))) eye(3)];

== matlab function PCwF2M/Kinematic Coordination/Manipulator Position//Orientation in World Frame ==
  data: p_do input; q_do input; x_d output; r parameter
function x_d = manipulatorpose(p_do,q_do,r)

x_d = [p_do + quatrot(q_do,r(1:3));
        %q_do;
        p_do + quatrot(q_do,r(4:6))];
        %q_do];
%         p_do + quatrot(q_do,r(7:9));
%         q_do;
%         p_do + quatrot(q_do,r(10:12));
%         q_do];

== matlab function PCwF2M/Kinematic Coordination/Centripetal Force ==
  data: dx_do input; b output; r parameter; q_do input
function b = centripetalforce(dx_do,r,q_do)
b = [skew_sm(dx_do(4:6))*skew_sm(dx_do(4:6))*quatrot(q_do,r(1:3));
     %zeros(3,1);
     skew_sm(dx_do(4:6))*skew_sm(dx_do(4:6))*quatrot(q_do,r(4:6))];
     %zeros(3,1)];
%      skew_sm(dx_do(4:6))*skew_sm(dx_do(4:6))*quatrot(x(4:7),r(7:9));
%      zeros(3,1);
%      skew_sm(dx_do(4:6))*skew_sm(dx_do(4:6))*quatrot(x(4:7),r(10:12));
%      zeros(3,1)];

== matlab function PCwF2M/Inverse Dynamics/MATLAB Function3 ==
  data: r parameter; G output; q_o input
function G = GraspMatrix(r,q_o)
%G = [eye(3) zeros(3) eye(3) zeros(3) eye(3) zeros(3) eye(3) zeros(3);
 %   skew_sm(quatrot(x(4:7),r(1:3))) eye(3) skew_sm(quatrot(x(4:7),r(4:6))) eye(3) skew_sm(quatrot(x(4:7),r(7:9))) eye(3) skew_sm(quatrot(x(4:7),r(10:12))) eye(3)];
 G = [eye(3) zeros(3) eye(3) zeros(3);
   skew_sm(quatrot(q_o,r(1:3))) eye(3) skew_sm(quatrot(q_o,r(4:6))) eye(3)];

== matlab function PCwF2M/Impedance control/Manipulator3/MATLAB Function2 ==
  data: eta3 input; K output; k3 parameter; kappa3 parameter
function K = stiffness(eta3,k3,kappa3)
K = blkdiag(k3*eye(3),2*eta3*kappa3*eye(3));

== matlab function PCwF2M/Impedance control/Manipulator4/MATLAB Function3 ==
  data: eta4 input; K output; k4 parameter; kappa4 parameter
function K = stiffness(eta4,k4,kappa4)
K = blkdiag(k4*eye(3),2*eta4*kappa4*eye(3));

== matlab function PCwF2M/Manipulator dynamics/Reduced Constraint Matrix ==
  data: r parameter; Ared output; x input
function Ared = ReducedConstraintMAtrix(r,x)
Ared = [-eye(3) skew_sm(quatrot(x(4:7),r(4:6)-r(1:3))) eye(3) zeros(3);
        zeros(3) -eye(3) zeros(3) eye(3) zeros(3,12)];
%         -eye(3) skew_sm(quatrot(x(4:7),r(7:9)-r(1:3))) zeros(3,6) eye(3) zeros(3,9);
%         zeros(3) -eye(3) zeros(3,9) eye(3) zeros(3,6);
%         -eye(3) skew_sm(quatrot(x(4:7),r(10:12)-r(1:3))) zeros(3,12) eye(3) zeros(3);
%         zeros(3) -eye(3) zeros(3,15) eye(3)];

== matlab function PCwF2M/Manipulator dynamics/Centripal Force ==
  data: r parameter; q_o input; bred output; dx_o input; ddx_o input
function bred = ReducedCentripetalvector(r,q_o,dx_o,ddx_o)
bred = [skew_sm(dx_o(4:6))*skew_sm(dx_o(4:6))*quatrot(q_o,(r(4:6)-r(1:3))) + skew_sm(quatrot(q_o,r(1:3))-quatrot(q_o,r(4:6)))*ddx_o(4:6)];
%         zeros(3,1);
%         skew_sm(dx(4:6))*skew_sm(dx(4:6))*quatrot(x(4:7),(r(7:9)-r(1:3)));
%         zeros(3,1);
%         skew_sm(dx(4:6))*skew_sm(dx(4:6))*quatrot(x(4:7),(r(10:12)-r(1:3)));
%         zeros(3,1)];

== matlab function PCwF2M/Interaction dynamics/Apparent Inertia ==
  data: G input; Mapp output; M input; m0 parameter; j0 parameter
function Mapp = ApparentInertia(G,M,m0,j0)
Mapp = blkdiag(m0*eye(3),j0*eye(3)) + G*M*G';

== matlab function PCwF2M/Interaction dynamics/Grasp Matrix ==
  data: r parameter; G output; x input
function G = GraspMatrix(r,x)
G = [eye(3) zeros(3) eye(3) zeros(3) eye(3) zeros(3) eye(3) zeros(3);
    skew_sm(quatrot(x(4:7),r(1:3))) eye(3) skew_sm(quatrot(x(4:7),r(4:6))) eye(3) skew_sm(quatrot(x(4:7),r(7:9))) eye(3) skew_sm(quatrot(x(4:7),r(10:12))) eye(3)];

== matlab function PCwF2M/Interaction dynamics/Coriolis Force ==
  data: dx input; hcoriolis output; j0 parameter; m0 parameter
function hcoriolis = CoriolisForce(dx,j0,m0)
hcoriolis = [m0*skew_sm(dx(4:6))*dx(1:3);
        j0*skew_sm(dx(4:6))*dx(4:6)];

== matlab function PCwF2M/Interaction dynamics/Centripetal Force ==
  data: dx input; b output; r parameter; x input
function b = centripetalforce(dx,r,x)
b = [skew_sm(dx(4:6))*skew_sm(dx(4:6))*quatrot(x(4:7),r(1:3));
     zeros(3,1);
     skew_sm(dx(4:6))*skew_sm(dx(4:6))*quatrot(x(4:7),r(4:6));
     zeros(3,1);
     skew_sm(dx(4:6))*skew_sm(dx(4:6))*quatrot(x(4:7),r(7:9));
     zeros(3,1);
     skew_sm(dx(4:6))*skew_sm(dx(4:6))*quatrot(x(4:7),r(10:12));
     zeros(3,1)];

== matlab function PCwF2M/Manipulator motion/Grasp Matrix ==
  data: r parameter; G output; q_o input
function G = GraspMatrix(r,q_o)
% G = [eye(3) zeros(3) eye(3) zeros(3) eye(3) zeros(3) eye(3) zeros(3);
%     skew_sm(quatrot(x(4:7),r(1:3))) eye(3) skew_sm(quatrot(x(4:7),r(4:6))) eye(3) skew_sm(quatrot(x(4:7),r(7:9))) eye(3) skew_sm(quatrot(x(4:7),r(10:12))) eye(3)];
G = [eye(3) zeros(3) eye(3) zeros(3);
    skew_sm(quatrot(q_o,r(1:3))) eye(3) skew_sm(quatrot(q_o,r(4:6))) eye(3)];

== matlab function PCwF2M/Manipulator motion/Manipualtor pose in world frame ==
  data: p_o input; q_o input size=4; x output; r parameter
function x = manipulatorpose(p_o,q_o,r)

x = [p_o + quatrot(q_o,r(1:3));
%         q_o;
        p_o + quatrot(q_o,r(4:6))];
%         q_o;
%         p_o + quatrot(q_o,r(7:9));
%         q_o;
%         p_o + quatrot(q_o,r(10:12));
%         q_o ];

== matlab function PCwF2M/Nullspace/Reduced Constraint Matrix ==
  data: r parameter; Ared output; x input
function Ared = ReducedConstraintMAtrix(r,x)
Ared = [-eye(3) skew_sm(quatrot(x(4:7),r(4:6)-r(1:3))) eye(3) zeros(3,15);
        zeros(3) -eye(3) zeros(3) eye(3) zeros(3,12);
        -eye(3) skew_sm(quatrot(x(4:7),r(7:9)-r(1:3))) zeros(3,6) eye(3) zeros(3,9);
        zeros(3) -eye(3) zeros(3,9) eye(3) zeros(3,6);
        -eye(3) skew_sm(quatrot(x(4:7),r(10:12)-r(1:3))) zeros(3,12) eye(3) zeros(3);
        zeros(3) -eye(3) zeros(3,15) eye(3)];

== matlab function PCwF2M/Allocator/MATLAB Function1 ==
  data: r parameter; bred output; dx input; x input
function bred = ReducedCentripetalvector(r,dx,x)
bred = [skew_sm(dx(4:6))*skew_sm(dx(4:6))*quatrot(x(4:7),r(4:6)-r(1:3));
    zeros(3,1);
    skew_sm(dx(4:6))*skew_sm(dx(4:6))*quatrot(x(4:7),r(7:9)-r(1:3));
    zeros(3,1);
    skew_sm(dx(4:6))*skew_sm(dx(4:6))*quatrot(x(4:7),r(10:12)-r(1:3));
    zeros(3,1)];

== matlab function PCwF2M/Allocator/MATLAB Function ==
  data: r parameter; Ared output; x input
function Ared = ReducedConstraintMAtrix(r,x)
Ared = [-eye(3) skew_sm(quatrot(x(4:7),r(4:6)-r(1:3))) eye(3) zeros(3,15);
        zeros(3) -eye(3) zeros(3) eye(3) zeros(3,12);
        -eye(3) skew_sm(quatrot(x(4:7),r(7:9)-r(1:3))) zeros(3,6) eye(3) zeros(3,9);
        zeros(3) -eye(3) zeros(3,9) eye(3) zeros(3,6);
        -eye(3) skew_sm(quatrot(x(4:7),r(10:12)-r(1:3))) zeros(3,12) eye(3) zeros(3);
        zeros(3) -eye(3) zeros(3,15) eye(3)];

== matlab function PCwF2M/Object to World Frame ==
  data: z input; x input; z_w output
function z_w = object2worldFrame(z,x)

z_w = [quatrot(x(4:7),z(1:3));
       z(4:6);
       quatrot(x(4:7),z(7:9));
       z(10:12);
       quatrot(x(4:7),z(13:15));
       z(16:18)];

== matlab function PCwF2M/Manipulator dynamics/World to Object Frame ==
  data: hw input; q_o input; h_int output
function h_int = inertial2objectFrame(hw,q_o)

% h_int = [quatrot(quatconj(x(4:7)')',hw(1:3));
%          hw(4:6);%quatrot(quatconj(x(4:7)')',hw(4:6));
%          quatrot(quatconj(x(4:7)')',hw(7:9));
%          hw(10:12);%quatrot(quatconj(x(4:7)')',hw(10:12));
%          quatrot(quatconj(x(4:7)')',hw(13:15));
%          hw(16:18);%quatrot(quatconj(x(4:7)')',hw(16:18));
%          quatrot(quatconj(x(4:7)')',hw(19:21));
%          hw(22:24)];%quatrot(quatconj(x(4:7)')',hw(22:24));];

h_int = [quatrot(quatconj(q_o')',hw(1:3));
         quatrot(quatconj(q_o')',hw(4:6))];
